simulink model "UAVLinCL_TRACK_ramp"  (R2023a)
settings: Solver=ode45  StartTime=0.0  StopTime=20  RelTol=1e-3  EnableMultiTasking=on
values from neighbouring files (symbols this model uses):
  A = [-0.5572,-0.7814;0.7814,0]    [Calculos02_Vnoladetrim.m]
  B = [1,-1;0,2]    [Calculos02_Vnoladetrim.m]
  C = [1.9691,6.4493]    [Calculos02_Vnoladetrim.m]
  Ct = [0, 0, 0, 0, 1]    [PI_6_Tracker_GS.m]    (also in PI_6_Tracker_bigGuy.m)
  K1 = Kt(:,1:5)    [PI_6_Tracker_GS.m]    (also in PI_6_Tracker_bigGuy.m)
  K2 = Kt(:,6)    [PI_6_Tracker_GS.m]    (also in PI_6_Tracker_bigGuy.m)
  x0t = zeros(5,1)    [PI_6_Tracker_GS.m]    (also in PI_6_Tracker_bigGuy.m)
undefined symbols (not defined in the file or in its folder): D, Utrim, Xtrim
libraries: simulink x2
settings Model: Creator=Ignacio  LastModifiedBy=ignac
settings SolverCC: AlgebraicLoopSolver=TrustRegion
settings DataIOCC: ExternalInput=[0 0.369809473744665 -0.0760167506859634 0.299999999999976]  InitialState=[]  LimitDataPoints=on  SaveFormat=Array  SignalLoggingSaveFormat=ModelDataLogs  ReturnWorkspaceOutputs=off
settings OptimizationCC: DefaultParameterBehavior=Inlined  BufferReuse=off  ExpressionDepthLimit=2147483647  LifeSpan=inf
settings DebuggingCC: UnderspecifiedInitializationDetection=Classic  MergeDetectMultiDrivingBlocksExec=none  FcnCallInpInsideContextMsg=warning  UnconnectedInputMsg=warning  UnconnectedOutputMsg=warning  UnconnectedLineMsg=warning  StateNameClashWarn=warning  InitInArrayFormatMsg=none  SFUnexpectedBacktrackingDiag=warning  SFNoUnconditionalDefaultTransitionDiag=warning  SFExecutionAtInitializationDiag=none  ArithmeticOperatorsInVariantConditions=warning
settings HardwareCC: ProdBitPerPointer=32  ProdBitPerSizeT=32  ProdBitPerPtrDiffT=32  ProdLargestAtomicFloat=None  ProdIntDivRoundTo=Undefined  ProdEndianess=Unspecified  ProdWordSize=32  ProdHWDeviceType=32-bit Generic
settings ModelReferenceCC: EnableRefExpFcnMdlSchedulingChecks=on  PropagateSignalLabelsOutOfModel=off
settings SFSimCC: SimUseLocalCustomCode=off  CustomCodeUndefinedFunction=UseInterfaceOnly
settings RTWCC: RTWUseLocalCustomCode=off
settings CodeAppCC: StateflowObjectComments=on
settings GRTTargetCC: TargetLangStandard=C89/C90 (ANSI)
settings ConfigComp: CovMetricSettings=dw  CovSaveCumulativeToWorkspaceVar=on  CovSaveSingleToWorkspaceVar=on  CovExternalEMLEnable=off

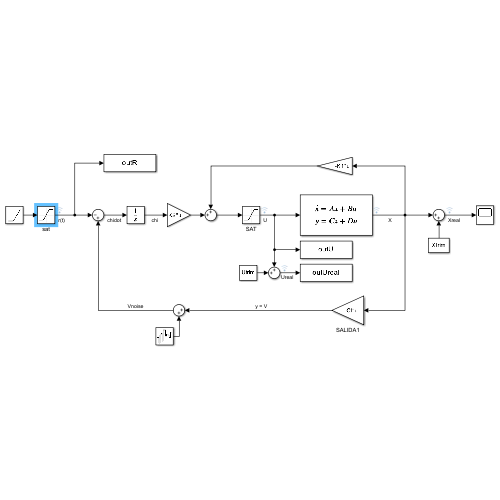
[thumbnail: Simulink's stored preview of the top-level diagram]
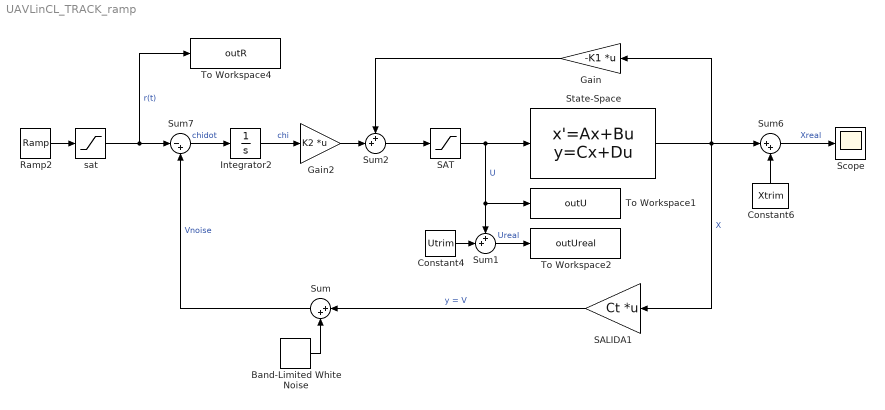
== system UAVLinCL_TRACK_ramp ==
  Band-Limited White Noise : simulink/Sources/Band-Limited White Noise  Cov=[0.1]*0  Ts=0.1  seed=[23341]
  Constant4 : Constant  Value=Utrim
  Constant6 : Constant  Value=Xtrim
  Gain : Gain  Gain=-K1  Multiplication=Matrix(K*u)
  Gain2 : Gain  Gain=K2  Multiplication=Matrix(K*u)
  Integrator2 : Integrator
  Ramp2 : simulink/Sources/Ramp  slope=1  start=0  InitialOutput=0
  SALIDA1 : Gain  Gain=Ct  Multiplication=Matrix(K*u)
  SAT : Saturate  UpperLimit=[1; 0.5] - Utrim  LowerLimit=[0; -0.5] - Utrim
  Scope : Scope
  State-Space : StateSpace  A=A  B=B  C=C  D=D  InitialCondition=x0t
  Sum : Sum  Inputs=|++
  Sum1 : Sum  Inputs=++|
  Sum2 : Sum  Inputs=++|
  Sum6 : Sum  Inputs=|++
  Sum7 : Sum  Inputs=|-+
  To Workspace1 : ToWorkspace  VariableName=outU  SampleTime=-1
      settings: Save2DSignal=2-D array (concatenate along first dimension)
  To Workspace2 : ToWorkspace  VariableName=outUreal  SampleTime=-1
      settings: Save2DSignal=2-D array (concatenate along first dimension)
  To Workspace4 : ToWorkspace  VariableName=outR  SampleTime=-1
      settings: Save2DSignal=2-D array (concatenate along first dimension)
  sat : Saturate  UpperLimit=10  LowerLimit=0
  wires:
  State-Space/1 -> SALIDA1/1, Sum6/1, Gain/1  "X"
  Band-Limited White Noise/1 -> Sum/2
  Constant6/1 -> Sum6/2
  SAT/1 -> To Workspace1/1, Sum1/1, State-Space/1  "U"
  SALIDA1/1 -> Sum/1  "y = V"
  Sum7/1 -> Integrator2/1  "chidot"
  Integrator2/1 -> Gain2/1  "chi"
  Sum/1 -> Sum7/2  "Vnoise"
  Gain2/1 -> Sum2/2
  Gain/1 -> Sum2/1
  Sum2/1 -> SAT/1
  Sum6/1 -> Scope/1  "Xreal"
  Sum1/1 -> To Workspace2/1  "Ureal"
  Constant4/1 -> Sum1/2
  Ramp2/1 -> sat/1
  sat/1 -> To Workspace4/1, Sum7/1  "r(t)"
